simulink model "mod_torque_con_PID_Obs"  (R2023b)
settings: Solver=VariableStepAuto  StartTime=0.0  StopTime=20  MaxStep=1e-4  MinStep=1e-6  RelTol=1e-2
values from neighbouring files (symbols this model uses):
  alpha_Cu = 3.9e-3    (= 0.0039)    [analisis_estabilidad.m]    (also in parametros.m; parametros_sim.m)
  b_a = 0.0396    [parametros.m]
  b_eq = b_eq_max    (= 2.40277777778e-05)    [analisis_estabilidad.m]    (also in parametros.m = 2.19444444444e-05; parametros_sim.m = 2.19444444444e-05)
  b_m = 15.0e-6    (= 1.5e-05)    [analisis_estabilidad.m]    (also in parametros.m; parametros_sim.m)
  C_ts = 0.818    [analisis_estabilidad.m]    (also in parametros.m; parametros_sim.m)
  g = 9.80665    [analisis_estabilidad.m]    (also in parametros.m; parametros_sim.m)
  J_eq = J_eq_max    (= 4.58263888889e-05)    [analisis_estabilidad.m]    (also in parametros.m = 1.97847222222e-05; parametros_sim.m = 1.97847222222e-05)
  J_m = 14.0e-6    (= 1.4e-05)    [analisis_estabilidad.m]    (also in parametros.m; parametros_sim.m)
  k_l = (m*l_cm + m_l*l_l)*g    (= 2.4516625)    [analisis_estabilidad.m]    (also in parametros.m = 0.25; parametros_sim.m)
  K_sa = 31.656    [parametros.m]
  K_sia = 10129.78    [parametros.m]
  L_d = 6.6    [analisis_estabilidad.m]    (also in parametros.m = 0.0066; parametros_sim.m; polosyceros.m = L_d^3)
  L_ls = 0.8    [analisis_estabilidad.m]    (also in parametros.m = 0.0008; parametros_sim.m)
  L_q = 5.8    [analisis_estabilidad.m]    (also in parametros.m = 0.0058; parametros_sim.m; polosyceros.m = L_q^3)
  lambda_m = 0.016    [analisis_estabilidad.m]    (also in parametros.m; parametros_sim.m)
  P_p = 3    [analisis_estabilidad.m]    (also in parametros.m; parametros_sim.m)
  r = 120    [analisis_estabilidad.m]    (also in parametros.m; parametros_sim.m)
  R_s_ref = 1.02    [analisis_estabilidad.m]    (also in parametros.m; parametros_sim.m)
  R_ts_amb = 146.7    [analisis_estabilidad.m]    (also in parametros.m; parametros_sim.m)
  T_s_ref = 20    [analisis_estabilidad.m]    (also in parametros.m; parametros_sim.m)
undefined symbols (not defined in the file or in its folder): Ke_i, Ke_o2, Ke_omega, Ke_t2, Ke_theta, sat, tau, wn_mod, wnc, wnt, z
libraries: SignalEditorBlockLib x4
settings Model: Creator=AAgus  LastModifiedBy=Marti
settings SolverCC: MaxConsecutiveMinStep=100

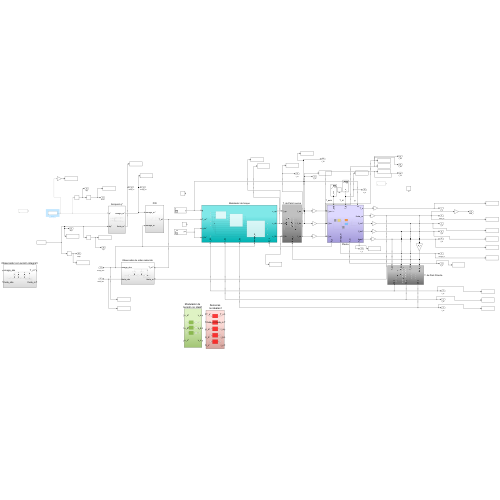
[thumbnail: Simulink's stored preview of the top-level diagram]
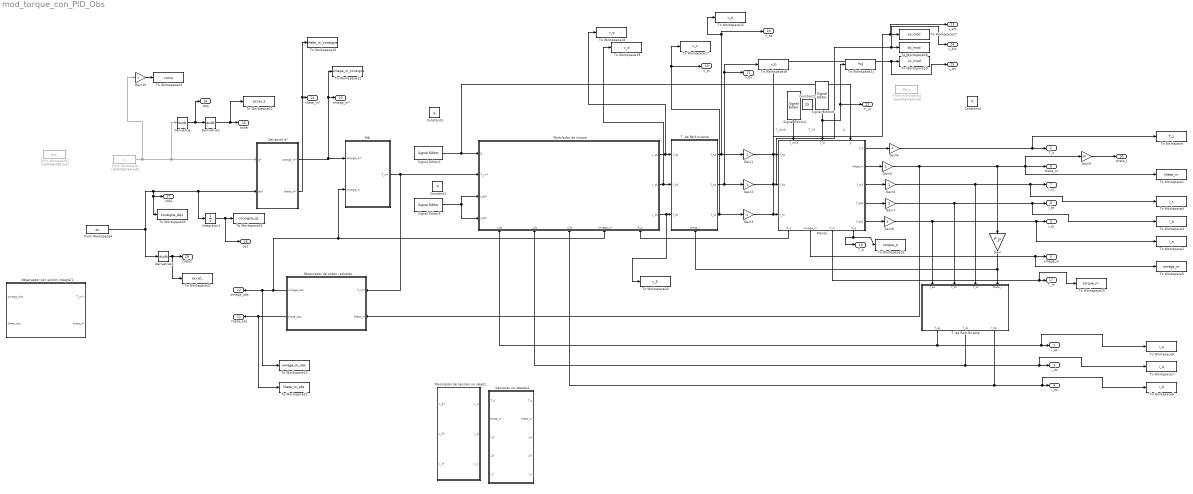
== system mod_torque_con_PID_Obs ==
  note: T_amb
  note: g
  note: T_ld
  Constant1 : Constant  Value=0
  Constant2 : Constant  Value=25
  Constant3 : Constant  Value=g
  Constant4 : Constant  Value=0
  Derivative : Derivative
  Derivative1 : Derivative
  Derivative3 : Derivative
  From Workspace : FromWorkspace  Commented=on  VariableName=u
  From Workspace1 : FromWorkspace  Commented=on  VariableName=duc
  From Workspace2 : FromWorkspace  Commented=on  VariableName=tld_c
  From Workspace4 : FromWorkspace  VariableName=du
  Gain : Gain  Gain=P_p
  Gain{1..8} (8 alike) : Gain
  Gain10 : Gain  Gain=r
  Gain9 : Gain  Gain=1/r
  Integrator1 : Integrator
  Modulador de tensión no ideal1 : Subsystem
  Modulador de torque : Subsystem
      settings: PortSchema="{\"entries\":[{\"content\":{\"sides\":[{\"content\":{\"connectorIds\":[\"In1\",\"In2\",\"In3\",\"In4\"]},\"type\":\"ConnectorPlacement.EquallySpacedRectSide\",\"uuid\":\"92ac8522-395f-4ce3-8f5e-792626a83240\"},{\"content\":{\"connectorIds\":[\"Out1\",\"Out2\",\"Out3\"],\"side\":\"RIGHT\"},\"type\":\"ConnectorPlacement.EquallySpacedRectSide\",\"uuid\":\"b1f2c717-a268-4393-91e6-df0d77a5b9df\"},{\"content\":{\"side\":\"TOP\"},\"type\":\"ConnectorPlacement.EquallySpacedRectSide\",\"uuid\":\"27380e77-d074-4889-aa22-28aab66abdda\"},{\"content\":{\"connectorIds\":[\"In5\",\"In6\",\"In7\",\"In8\",\"In9\"],\"side\":\"BOTTOM\"},\"type\":\"ConnectorPlacement.EquallySpacedRectSide\",\"uuid\":\"8a4427a4-2d74-404b-8b0d-69ab3b710b0e\"}]},\"type\":\"ConnectorPlacement.EquallySpacedConnector\",\"uuid\":\"19c0cced-0884-4633-8ad3-2d6d5d480879\"}],\"packageUris\":[\"http://schema.mathworks.com/mf0/Connector/R2020b\"],\"version\":\"1.0\"}"
  Observador con acción integral1 : Subsystem
      settings: PortSchema="{\"entries\":[{\"content\":{\"sides\":[{\"content\":{\"connectorIds\":[\"Out1\",\"Out2\"]},\"type\":\"ConnectorPlacement.EquallySpacedRectSide\",\"uuid\":\"7f1ab875-1cda-4cac-85ff-ce07181c17e4\"},{\"content\":{\"connectorIds\":[\"In1\",\"In2\"],\"side\":\"RIGHT\"},\"type\":\"ConnectorPlacement.EquallySpacedRectSide\",\"uuid\":\"6b91254d-cc96-42c9-a758-369a40099a6f\"},{\"content\":{\"side\":\"TOP\"},\"type\":\"ConnectorPlacement.EquallySpacedRectSide\",\"uuid\":\"4cd12954-6c23-434d-8bef-175e9edf0377\"}]},\"type\":\"ConnectorPlacement.EquallySpacedConnector\",\"uuid\":\"b17f3470-00fb-4a2f-9925-fdd3ec829801\"}],\"packageUris\":[\"http://schema.mathworks.com/mf0/Connector/R2020b\"],\"version\":\"1.0\"}"
  Observador de orden reducido : Subsystem
  PID : Subsystem
  Planta : Subsystem
      settings: PortSchema="{\"entries\":[{\"content\":{\"sides\":[{\"content\":{\"connectorIds\":[\"In1\",\"In2\",\"In3\"]},\"type\":\"ConnectorPlacement.EquallySpacedRectSide\",\"uuid\":\"9ff39df0-8326-46b1-b650-24ffd78ea64a\"},{\"content\":{\"connectorIds\":[\"Out1\",\"Out2\",\"Out3\",\"Out4\",\"Out5\"],\"side\":\"RIGHT\"},\"type\":\"ConnectorPlacement.EquallySpacedRectSide\",\"uuid\":\"3d3bc9f1-e392-438d-8ee1-0a3eb241c21d\"},{\"content\":{\"connectorIds\":[\"In4\",\"In5\",\"In6\"],\"side\":\"TOP\"},\"type\":\"ConnectorPlacement.EquallySpacedRectSide\",\"uuid\":\"c4910fb7-2fb9-4a3e-8c96-07515026454c\"},{\"content\":{\"connectorIds\":[\"Out6\",\"Out7\",\"Out8\",\"Out9\"],\"side\":\"BOTTOM\"},\"type\":\"ConnectorPlacement.EquallySpacedRectSide\",\"uuid\":\"63ebca1e-77c7-4a83-9d7f-f511e7e06496\"}]},\"type\":\"ConnectorPlacement.EquallySpacedConnector\",\"uuid\":\"6053906f-09a1-4145-a7f8-0fc1307cd3c1\"}],\"packageUris\":[\"http://schema.mathworks.com/mf0/Connector/R2020b\"],\"version\":\"1.0\"}"
  Sensores no ideales1 : Subsystem
  Set-point q* : Subsystem
  Signal Editor2 : SignalEditorBlockLib/Signal Editor  FileName=gravedad.mat  ActiveScenario=g  ActiveSignal=g  IsBus=off  OutputBusObjectStr=Bus: BusObject  SampleTime=0  Interpolate=off  ZeroCross=off  OutputAfterFinalValue=Setting to zero  Unit=inherit  PreserveSignalName=on  ApplySigPropsToAllScenarios=on  ApplySigPropsToAllSignals=off
  Signal Editor4 : SignalEditorBlockLib/Signal Editor  FileName=tamb.mat  ActiveScenario=T_amb  ActiveSignal=T_amb  IsBus=off  OutputBusObjectStr=Bus: BusObject  SampleTime=0  Interpolate=off  ZeroCross=off  OutputAfterFinalValue=Setting to zero  Unit=inherit  PreserveSignalName=on  ApplySigPropsToAllScenarios=on  ApplySigPropsToAllSignals=off
  Signal Editor5 : SignalEditorBlockLib/Signal Editor  FileName=corrientes_d0.mat  ActiveScenario=i_d0  ActiveSignal=i_d0  IsBus=off  OutputBusObjectStr=Bus: BusObject  SampleTime=0  Interpolate=off  ZeroCross=off  OutputAfterFinalValue=Setting to zero  Unit=inherit  PreserveSignalName=on  ApplySigPropsToAllScenarios=on  ApplySigPropsToAllSignals=off
  Signal Editor6 : SignalEditorBlockLib/Signal Editor  FileName=T_ld.mat  ActiveScenario=T_ld  ActiveSignal=T_ld  IsBus=off  OutputBusObjectStr=Bus: BusObject  SampleTime=0  Interpolate=off  ZeroCross=off  OutputAfterFinalValue=Setting to zero  Unit=inherit  PreserveSignalName=on  ApplySigPropsToAllScenarios=on  ApplySigPropsToAllSignals=off
  T. de Park Directa : Subsystem
  T. de Park Inversa : Subsystem
      settings: PortSchema="{\"entries\":[{\"content\":{\"sides\":[{\"content\":{\"connectorIds\":[\"In1\",\"In2\",\"In3\"]},\"type\":\"ConnectorPlacement.EquallySpacedRectSide\",\"uuid\":\"87a6b8c1-3fd8-4d15-81b7-6d19a59b6fe3\"},{\"content\":{\"connectorIds\":[\"Out1\",\"Out2\",\"Out3\"],\"side\":\"RIGHT\"},\"type\":\"ConnectorPlacement.EquallySpacedRectSide\",\"uuid\":\"ab7c1476-3519-4f3e-a604-adca334ac53f\"},{\"content\":{\"side\":\"TOP\"},\"type\":\"ConnectorPlacement.EquallySpacedRectSide\",\"uuid\":\"325a5f4a-a59c-4f4e-a8f9-a592ceecf271\"},{\"content\":{\"connectorIds\":[\"In4\"],\"side\":\"BOTTOM\"},\"type\":\"ConnectorPlacement.EquallySpacedRectSide\",\"uuid\":\"c8952c47-ee5f-4725-8e8a-36e5b1bf9c18\"}]},\"type\":\"ConnectorPlacement.EquallySpacedConnector\",\"uuid\":\"8a5a5c71-0ab4-4571-9e71-296ad9f443dc\"}],\"packageUris\":[\"http://schema.mathworks.com/mf0/Connector/R2020b\"],\"version\":\"1.0\"}"
  To Workspace : ToWorkspace  VariableName=T_s  SaveFormat=Timeseries  SampleTime=-1
  To Workspace1 : ToWorkspace  VariableName=theta_m  SaveFormat=Timeseries  SampleTime=-1
  To Workspace10 : ToWorkspace  VariableName=theta_m_consigna  SaveFormat=Timeseries  SampleTime=-1
  To Workspace11 : ToWorkspace  VariableName=omega_m_consigna  SaveFormat=Timeseries  SampleTime=-1
  To Workspace12 : ToWorkspace  VariableName=theta_m_obs  SaveFormat=Timeseries  SampleTime=-1
  To Workspace13 : ToWorkspace  VariableName=omega_m_obs  SaveFormat=Timeseries  SampleTime=-1
  To Workspace15 : ToWorkspace  VariableName=v_a  SaveFormat=Timeseries  SampleTime=-1
  To Workspace16 : ToWorkspace  VariableName=v_b  SaveFormat=Timeseries  SampleTime=-1
  To Workspace17 : ToWorkspace  VariableName=v_c  SaveFormat=Timeseries  SampleTime=-1
  To Workspace18 : ToWorkspace  VariableName=v_q  SaveFormat=Timeseries  SampleTime=-1
  To Workspace19 : ToWorkspace  VariableName=v_d  SaveFormat=Timeseries  SampleTime=-1
  To Workspace2 : ToWorkspace  VariableName=i_a  SaveFormat=Timeseries  SampleTime=-1
  To Workspace20 : ToWorkspace  VariableName=v_0  SaveFormat=Timeseries  SampleTime=-1
  To Workspace21 : ToWorkspace  VariableName=Tld  SaveFormat=Timeseries  SampleTime=-1
  To Workspace22 : ToWorkspace  VariableName=accel_1  SaveFormat=Timeseries  SampleTime=-1
  To Workspace24 : ToWorkspace  VariableName=comp  SaveFormat=Timeseries  SampleTime=-1
  To Workspace25 : ToWorkspace  VariableName=torque_m  SaveFormat=Timeseries  SampleTime=-1
  To Workspace26 : ToWorkspace  VariableName=torque_q  SaveFormat=Timeseries  SampleTime=-1
  To Workspace27 : ToWorkspace  VariableName=va_mod  SaveFormat=Timeseries  SampleTime=-1
  To Workspace28 : ToWorkspace  VariableName=vb_mod  SaveFormat=Timeseries  SampleTime=-1
  To Workspace29 : ToWorkspace  VariableName=vc_mod  SaveFormat=Timeseries  SampleTime=-1
  To Workspace3 : ToWorkspace  VariableName=i_b  SaveFormat=Timeseries  SampleTime=-1
  To Workspace30 : ToWorkspace  VariableName=consigna_dq1  SaveFormat=Timeseries  SampleTime=-1
  To Workspace31 : ToWorkspace  VariableName=accel_  SaveFormat=Timeseries  SampleTime=-1
  To Workspace32 : ToWorkspace  VariableName=consigna_q1  SaveFormat=Timeseries  SampleTime=-1
  To Workspace4 : ToWorkspace  VariableName=i_c  SaveFormat=Timeseries  SampleTime=-1
  To Workspace5 : ToWorkspace  VariableName=omega_m  SaveFormat=Timeseries  SampleTime=-1
  To Workspace6 : ToWorkspace  VariableName=i_0  SaveFormat=Timeseries  SampleTime=-1
  To Workspace7 : ToWorkspace  VariableName=i_d  SaveFormat=Timeseries  SampleTime=-1
  To Workspace8 : ToWorkspace  VariableName=i_q  SaveFormat=Timeseries  SampleTime=-1
  T_s : Outport
  i_qs : Outport  Port=2
  i_ds : Outport  Port=3
  i_0s : Outport  Port=4
  omega_m : Outport  Port=5
  theta_m : Outport  Port=6
  i_cs : Outport  Port=7
  i_bs : Outport  Port=8
  i_as : Outport  Port=9
  theta_l : Outport  Port=10
  theta_obs : Outport  Port=11
  omega_obs : Outport  Port=12
  omega_m* : Outport  Port=13
  theta_m* : Outport  Port=14
  accel : Outport  Port=15
  dqq : Outport  Port=16
  T_m : Outport  Port=17
  T_q : Outport  Port=18
  v_cs : Outport  Port=19
  v_as : Outport  Port=20
  v_bs : Outport  Port=21
  T_ld : Outport  Port=22
  v_am : Outport  Port=23
  v_bm : Outport  Port=24
  v_cm : Outport  Port=25
  cq1 : Outport  Port=26
  cdq1 : Outport  Port=27
  cddq1 : Outport  Port=28
  wires:
  Gain9/1 -> theta_l/1
  Gain7/1 -> To Workspace3/1, i_bs/1, T. de Park Directa/2(f_bs)
  Planta/2(theta_m) -> Gain5/1
  Signal Editor2/1 -> Modulador de torque/1(g), Planta/6(g)
  T. de Park Inversa/3(f_cs) -> Gain3/1, v_cs/1, To Workspace17/1
  Gain6/1 -> T. de Park Directa/3(f_cs), To Workspace4/1, i_cs/1
  Signal Editor4/1 -> Planta/4(T_amb)
  T. de Park Directa/2(f_ds) -> Modulador de torque/6(i_ds), To Workspace7/1, i_ds/1
  T. de Park Inversa/1(f_as) -> Gain1/1, v_as/1, To Workspace15/1
  Planta/4(f_bs1) -> Gain7/1
  T. de Park Directa/3(f_0s) -> To Workspace6/1, i_0s/1, Modulador de torque/7(i_0s)
  Planta/7(omega_m) -> To Workspace5/1, omega_m/1
  Gain4/1 -> To Workspace/1, T_s/1
  T. de Park Directa/1(f_qs) -> To Workspace8/1, i_qs/1, Modulador de torque/5(i_qs)
  T. de Park Inversa/2(f_bs) -> Gain2/1, To Workspace16/1, v_bs/1
  Gain5/1 -> Observador de orden reducido/2(theta_m), To Workspace1/1, Gain9/1, theta_m/1, Gain/1
  Planta/1(T_s) -> Gain4/1
  Gain8/1 -> To Workspace2/1, i_as/1, T. de Park Directa/1(f_as)
  Planta/3(f_cs1) -> Gain6/1
  Gain/1 -> T. de Park Directa/4(theta_r), T. de Park Inversa/4(theta_r)
  Planta/5(f_as1) -> Gain8/1
  Modulador de torque/1(v_qs) -> To Workspace18/1, T. de Park Inversa/1(f_qs)
  Modulador de torque/2(v_ds) -> To Workspace19/1, T. de Park Inversa/2(f_ds)
  Modulador de torque/3(v_0s) -> To Workspace20/1, T. de Park Inversa/3(f_0s)
  Planta/6(R_s) -> Modulador de torque/9(R_s)
  Signal Editor5/1 -> Modulador de torque/3(i_ds*), Modulador de torque/4(i_0s*)
  PID/1(T_m*) -> Observador de orden reducido/1(T_m'*), Modulador de torque/2(T_m'*)
  Set-point q*/1(omega_m*) -> omega_m*/1, To Workspace11/1, PID/1(omega_m*)
  Observador de orden reducido/2(theta_obs) -> To Workspace12/1, theta_obs/1
  Observador de orden reducido/1(omega_obs) -> PID/2(omega_m), Modulador de torque/8(omega_m), To Workspace13/1, omega_obs/1
  Set-point q*/2(theta_m*) -> To Workspace10/1, theta_m*/1
  From Workspace/1 -> Gain10/1, Derivative/1, Set-point q*/1(q*)
  Derivative/1 -> dqq/1, Derivative1/1
  Derivative1/1 -> To Workspace22/1, accel/1
  Gain10/1 -> To Workspace24/1
  Planta/8(T_m) -> To Workspace25/1, T_m/1
  Planta/9(T_q) -> T_q/1, To Workspace26/1
  Signal Editor6/1 -> To Workspace21/1, T_ld/1, Planta/5(T_ld)
  Gain1/1 -> v_am/1, To Workspace27/1, Planta/1(f_as)
  Gain2/1 -> v_bm/1, To Workspace28/1, Planta/2(f_bs)
  Gain3/1 -> v_cm/1, To Workspace29/1, Planta/3(f_cs)
  Derivative3/1 -> cddq1/1, To Workspace31/1
  Integrator1/1 -> To Workspace32/1, cq1/1
  From Workspace4/1 -> Derivative3/1, cdq1/1, To Workspace30/1, Set-point q*/2(dq*), Integrator1/1

== system mod_torque_con_PID_Obs/Modulador de tensión no ideal1 ==
  v_a* : Inport
  v_b* : Inport  Port=2
  v_c* : Inport  Port=3
  A : Subsystem
  B : Subsystem
  C : Subsystem
  Saturation3 : Saturate  UpperLimit=sat  LowerLimit=-sat
  Saturation4 : Saturate  UpperLimit=sat  LowerLimit=-sat
  Saturation5 : Saturate  UpperLimit=sat  LowerLimit=-sat
  v_a : Outport
  v_b : Outport  Port=2
  v_c : Outport  Port=3
  wires:
  Saturation5/1 -> v_c/1
  Saturation4/1 -> v_b/1
  Saturation3/1 -> v_a/1
  C/1(v_c) -> Saturation5/1
  B/1(v_b) -> Saturation4/1
  A/1(v_a) -> Saturation3/1
  v_b*/1 -> B/1(v_b*)
  v_a*/1 -> A/1(v_a*)
  v_c*/1 -> C/1(v_c*)

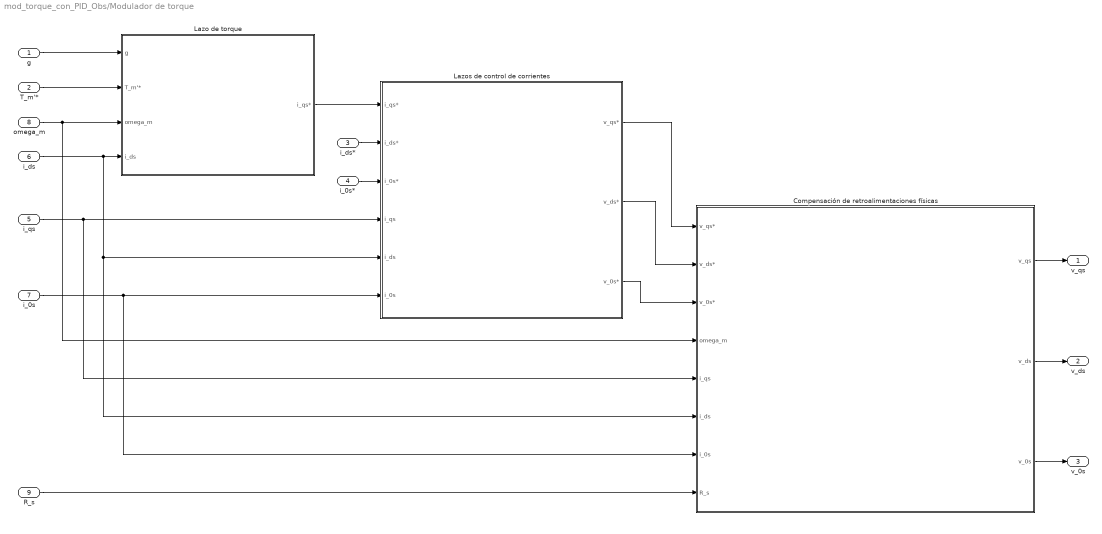
== system mod_torque_con_PID_Obs/Modulador de torque ==
  g : Inport
  T_m'* : Inport  Port=2
  i_ds* : Inport  Port=3
  i_0s* : Inport  Port=4
  i_qs : Inport  Port=5
  i_ds : Inport  Port=6
  i_0s : Inport  Port=7
  omega_m : Inport  Port=8
  R_s : Inport  Port=9
  Compensación de retroalimentaciones físicas : Subsystem
  Lazo de torque : Subsystem
  Lazos de control de corrientes : Subsystem
  v_qs : Outport
  v_ds : Outport  Port=2
  v_0s : Outport  Port=3
  wires:
  Lazos de control de corrientes/3(v_0s*) -> Compensación de retroalimentaciones físicas/3(v_0s*)
  i_ds*/1 -> Lazos de control de corrientes/2(i_ds*)
  T_m'*/1 -> Lazo de torque/2(T_m'*)
  Lazos de control de corrientes/1(v_qs*) -> Compensación de retroalimentaciones físicas/1(v_qs*)
  Lazos de control de corrientes/2(v_ds*) -> Compensación de retroalimentaciones físicas/2(v_ds*)
  omega_m/1 -> Lazo de torque/3(omega_m), Compensación de retroalimentaciones físicas/4(omega_m)
  Lazo de torque/1(i_qs*) -> Lazos de control de corrientes/1(i_qs*)
  g/1 -> Lazo de torque/1(g)
  Compensación de retroalimentaciones físicas/3(v_0s) -> v_0s/1
  i_ds/1 -> Compensación de retroalimentaciones físicas/6(i_ds), Lazos de control de corrientes/5(i_ds), Lazo de torque/4(i_ds)
  Compensación de retroalimentaciones físicas/1(v_qs) -> v_qs/1
  i_0s*/1 -> Lazos de control de corrientes/3(i_0s*)
  Compensación de retroalimentaciones físicas/2(v_ds) -> v_ds/1
  i_qs/1 -> Compensación de retroalimentaciones físicas/5(i_qs), Lazos de control de corrientes/4(i_qs)
  i_0s/1 -> Compensación de retroalimentaciones físicas/7(i_0s), Lazos de control de corrientes/6(i_0s)
  R_s/1 -> Compensación de retroalimentaciones físicas/8(R_s)

== system mod_torque_con_PID_Obs/Observador con acción integral1 ==
  note: e_theta
  T_m'* : Inport
  theta_m : Inport  Port=2
  Gain : Gain  Gain=1/J_eq
  Gain1 : Gain  Gain=Ke_o2
  Gain2 : Gain  Gain=Ke_i
  Gain3 : Gain  Gain=Ke_t2
  Integrator : Integrator
  Integrator1 : Integrator
  Integrator2 : Integrator
  Sum : Sum  Inputs=++|
  Sum1 : Sum  Inputs=++|
  Sum2 : Sum  Inputs=++|
  Sum3 : Sum  Inputs=+-
  omega_obs : Outport
  theta_obs : Outport  Port=2
  wires:
  Integrator/1 -> Sum2/2
  Sum/1 -> Sum1/2
  Gain1/1 -> Sum1/1
  Integrator2/1 -> Gain2/1
  Gain3/1 -> Sum2/1
  Sum2/1 -> Integrator1/1, omega_obs/1
  Integrator1/1 -> Sum3/2, theta_obs/1
  Gain2/1 -> Sum/1
  theta_m/1 -> Sum3/1
  T_m'*/1 -> Gain/1
  Gain/1 -> Sum/2
  Sum3/1 -> Gain3/1, Gain1/1, Integrator2/1
  Sum1/1 -> Integrator/1

== system mod_torque_con_PID_Obs/Observador de orden reducido ==
  note: e_theta
  T_m'* : Inport
  theta_m : Inport  Port=2
  Gain : Gain  Gain=1/J_eq
  Gain1 : Gain  Gain=Ke_omega
  Gain6 : Gain  Gain=Ke_theta
  Integrator : Integrator
  Integrator1 : Integrator
  Sum1 : Sum  Inputs=++|
  Sum3 : Sum  Inputs=++|
  Sum6 : Sum  Inputs=+-
  omega_obs : Outport
  theta_obs : Outport  Port=2
  wires:
  Gain/1 -> Sum1/2
  Sum1/1 -> Integrator/1
  Integrator1/1 -> theta_obs/1, Sum6/2
  theta_m/1 -> Sum6/1
  Gain6/1 -> Sum3/1
  Gain1/1 -> Sum1/1
  Sum6/1 -> Gain1/1, Gain6/1
  Sum3/1 -> omega_obs/1, Integrator1/1
  T_m'*/1 -> Gain/1
  Integrator/1 -> Sum3/2

== system mod_torque_con_PID_Obs/PID ==
  note: e_theta
  note: e_omega
  note: e_theta
  note: e_omega
  note: I
  note: P
  note: D
  omega_m* : Inport
  omega_m : Inport  Port=2
  Gain : Gain  Gain=K_sia
  Gain1 : Gain  Gain=K_sa
  Gain2 : Gain  Gain=b_a
  Integrator : Integrator
  Integrator1 : Integrator
  Sum : Sum  Inputs=|+-
  Sum1 : Sum  Inputs=+++
  T_m* : Outport
  wires:
  Gain2/1 -> Sum1/3
  Gain1/1 -> Sum1/2
  Integrator1/1 -> Gain1/1, Integrator/1
  Sum1/1 -> T_m*/1
  omega_m/1 -> Sum/2
  Gain/1 -> Sum1/1
  Integrator/1 -> Gain/1
  omega_m*/1 -> Sum/1
  Sum/1 -> Gain2/1, Integrator1/1

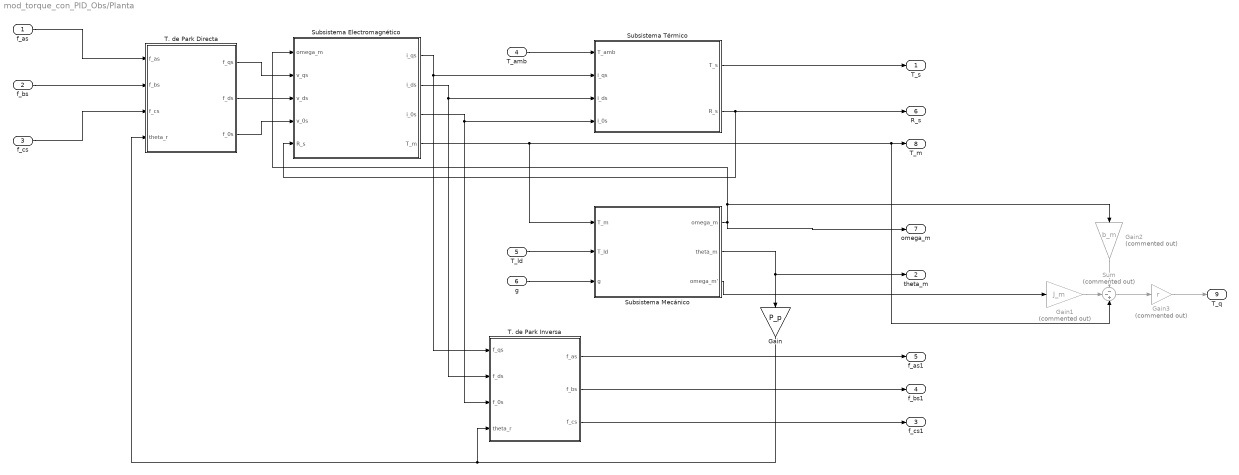
== system mod_torque_con_PID_Obs/Planta ==
  f_as : Inport
  f_bs : Inport  Port=2
  f_cs : Inport  Port=3
  T_amb : Inport  Port=4
  T_ld : Inport  Port=5
  g : Inport  Port=6
  Gain : Gain  Gain=P_p
  Gain1 : Gain  Commented=on  Gain=J_m
  Gain2 : Gain  Commented=on  Gain=b_m
  Gain3 : Gain  Commented=on  Gain=r
  Subsistema Electromagnético : Subsystem
  Subsistema Mecánico : Subsystem
  Subsistema Térmico : Subsystem
  Sum : Sum  Commented=on  Inputs=--+
  T. de Park Directa : Subsystem
  T. de Park Inversa : Subsystem
  T_s : Outport
  theta_m : Outport  Port=2
  f_cs1 : Outport  Port=3
  f_bs1 : Outport  Port=4
  f_as1 : Outport  Port=5
  R_s : Outport  Port=6
  omega_m : Outport  Port=7
  T_m : Outport  Port=8
  T_q : Outport  Port=9
  wires:
  f_as/1 -> T. de Park Directa/1(f_as)
  T. de Park Directa/1(f_qs) -> Subsistema Electromagnético/2(v_qs)
  T. de Park Directa/3(f_0s) -> Subsistema Electromagnético/4(v_0s)
  Subsistema Térmico/1(T_s) -> T_s/1
  T. de Park Inversa/1(f_as) -> f_as1/1
  T_amb/1 -> Subsistema Térmico/1(T_amb)
  Subsistema Electromagnético/3(i_0s) -> T. de Park Inversa/3(f_0s), Subsistema Térmico/4(i_0s)
  f_bs/1 -> T. de Park Directa/2(f_bs)
  T_ld/1 -> Subsistema Mecánico/2(T_ld)
  T. de Park Inversa/3(f_cs) -> f_cs1/1
  f_cs/1 -> T. de Park Directa/3(f_cs)
  T. de Park Inversa/2(f_bs) -> f_bs1/1
  Gain/1 -> T. de Park Directa/4(theta_r), T. de Park Inversa/4(theta_r)
  T. de Park Directa/2(f_ds) -> Subsistema Electromagnético/3(v_ds)
  Subsistema Térmico/2(R_s) -> Subsistema Electromagnético/5(R_s), R_s/1
  Subsistema Electromagnético/2(i_ds) -> T. de Park Inversa/2(f_ds), Subsistema Térmico/3(i_ds)
  Subsistema Electromagnético/1(i_qs) -> T. de Park Inversa/1(f_qs), Subsistema Térmico/2(i_qs)
  Subsistema Electromagnético/4(T_m) -> Sum/3, T_m/1, Subsistema Mecánico/1(T_m)
  Subsistema Mecánico/1(omega_m) -> omega_m/1, Gain2/1, Subsistema Electromagnético/1(omega_m)
  Subsistema Mecánico/2(theta_m) -> Gain/1, theta_m/1
  g/1 -> Subsistema Mecánico/3(g)
  Subsistema Mecánico/3(omega_m') -> Gain1/1
  Gain1/1 -> Sum/2
  Gain2/1 -> Sum/1
  Sum/1 -> Gain3/1
  Gain3/1 -> T_q/1

== system mod_torque_con_PID_Obs/Sensores no ideales1 ==
  T_s' : Inport
  theta_m' : Inport  Port=2
  i_a' : Inport  Port=3
  i_b' : Inport  Port=4
  i_c' : Inport  Port=5
  Sensor de Corriente A : Subsystem
  Sensor de Corriente B : Subsystem
  Sensor de Corriente C : Subsystem
  Sensor de Posición : Subsystem
  Sensor de Temperatura : Subsystem
  T_s : Outport
  theta_m : Outport  Port=2
  i_a : Outport  Port=3
  i_b : Outport  Port=4
  i_c : Outport  Port=5
  wires:
  i_c'/1 -> Sensor de Corriente C/1(i_c')
  i_b'/1 -> Sensor de Corriente B/1(i_b')
  Sensor de Corriente C/1(i_c) -> i_c/1
  Sensor de Temperatura/1(T_s) -> T_s/1
  theta_m'/1 -> Sensor de Posición/1(theta_m')
  i_a'/1 -> Sensor de Corriente A/1(i_a')
  Sensor de Corriente B/1(i_b) -> i_b/1
  Sensor de Posición/1(theta_m) -> theta_m/1
  T_s'/1 -> Sensor de Temperatura/1(T_s')
  Sensor de Corriente A/1(i_a) -> i_a/1

== system mod_torque_con_PID_Obs/Set-point q* ==
  q* : Inport
  dq* : Inport  Port=2
  Derivative : Derivative
  Gain1 : Gain  Gain=r
  Gain11 : Gain  Gain=r
  Integrator : Integrator
  Manual Switch : ManualSwitch  CurrentSetting=0
  Manual Switch1 : ManualSwitch  CurrentSetting=0
  omega_m* : Outport
  theta_m* : Outport  Port=2
  wires:
  q*/1 -> Gain11/1
  Gain11/1 -> Manual Switch/1, Derivative/1
  Manual Switch/1 -> theta_m*/1
  dq*/1 -> Gain1/1
  Manual Switch1/1 -> omega_m*/1
  Gain1/1 -> Manual Switch1/2, Integrator/1
  Derivative/1 -> Manual Switch1/1
  Integrator/1 -> Manual Switch/2

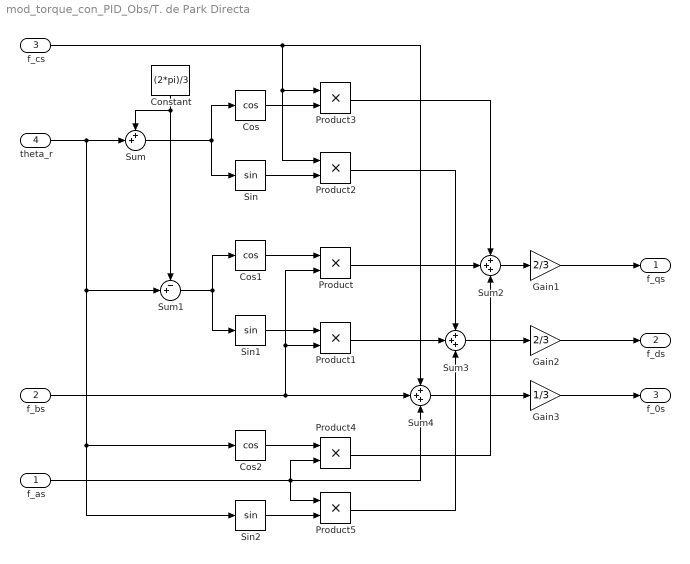
== system mod_torque_con_PID_Obs/T. de Park Directa ==
  f_as : Inport
  f_bs : Inport  Port=2
  f_cs : Inport  Port=3
  theta_r : Inport  Port=4
  Constant : Constant  Value=(2*pi)/3
  Cos : Trigonometry  Operator=cos
  Cos1 : Trigonometry  Operator=cos
  Cos2 : Trigonometry  Operator=cos
  Gain1 : Gain  Gain=2/3
  Gain2 : Gain  Gain=2/3
  Gain3 : Gain  Gain=1/3
  Product{,1..5} (6 alike) : Product
  Sin : Trigonometry
  Sin1 : Trigonometry
  Sin2 : Trigonometry
  Sum : Sum  Inputs=++|
  Sum1 : Sum  Inputs=-+|
  Sum2 : Sum  Inputs=+++
  Sum3 : Sum  Inputs=+++
  Sum4 : Sum  Inputs=+++
  f_qs : Outport
  f_ds : Outport  Port=2
  f_0s : Outport  Port=3
  wires:
  Product4/1 -> Sum2/3
  Cos1/1 -> Product/1
  theta_r/1 -> Sum/2, Sin2/1, Cos2/1, Sum1/2
  Sin1/1 -> Product1/1
  Sin2/1 -> Product5/2
  Product3/1 -> Sum2/1
  Cos2/1 -> Product4/1
  Product1/1 -> Sum3/2
  f_as/1 -> Sum4/3, Product4/2, Product5/1
  Sum2/1 -> Gain1/1
  Sum1/1 -> Sin1/1, Cos1/1
  f_bs/1 -> Sum4/2, Product/2, Product1/2
  Sum/1 -> Sin/1, Cos/1
  Product2/1 -> Sum3/1
  Sin/1 -> Product2/2
  Sum4/1 -> Gain3/1
  Gain1/1 -> f_qs/1
  f_cs/1 -> Sum4/1, Product2/1, Product3/1
  Gain2/1 -> f_ds/1
  Product/1 -> Sum2/2
  Sum3/1 -> Gain2/1
  Cos/1 -> Product3/2
  Constant/1 -> Sum1/1, Sum/1
  Gain3/1 -> f_0s/1
  Product5/1 -> Sum3/3

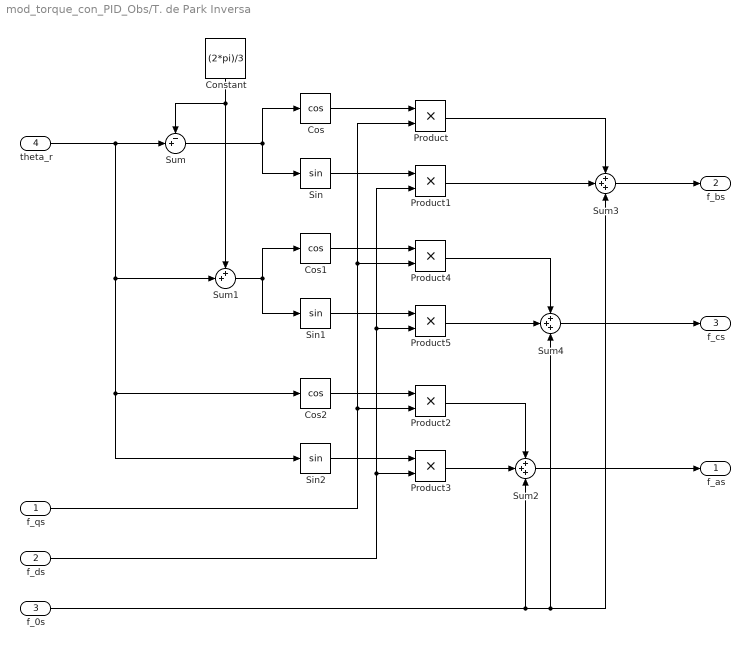
== system mod_torque_con_PID_Obs/T. de Park Inversa ==
  f_qs : Inport
  f_ds : Inport  Port=2
  f_0s : Inport  Port=3
  theta_r : Inport  Port=4
  Constant : Constant  Value=(2*pi)/3
  Cos : Trigonometry  Operator=cos
  Cos1 : Trigonometry  Operator=cos
  Cos2 : Trigonometry  Operator=cos
  Product{,1..5} (6 alike) : Product
  Sin : Trigonometry
  Sin1 : Trigonometry
  Sin2 : Trigonometry
  Sum : Sum  Inputs=-+|
  Sum1 : Sum  Inputs=++|
  Sum2 : Sum  Inputs=+++
  Sum3 : Sum  Inputs=+++
  Sum4 : Sum  Inputs=+++
  f_as : Outport
  f_bs : Outport  Port=2
  f_cs : Outport  Port=3
  wires:
  Product4/1 -> Sum4/1
  Sum2/1 -> f_as/1
  f_qs/1 -> Product4/2, Product/2, Product2/2
  Sum/1 -> Sin/1, Cos/1
  theta_r/1 -> Sum1/2, Cos2/1, Sin2/1, Sum/2
  Product1/1 -> Sum3/2
  Product3/1 -> Sum2/2
  Product5/1 -> Sum4/2
  Sin1/1 -> Product5/1
  Product/1 -> Sum3/1
  Cos/1 -> Product/1
  Sin2/1 -> Product3/1
  Cos1/1 -> Product4/1
  Sin/1 -> Product1/1
  f_0s/1 -> Sum3/3, Sum4/3, Sum2/3
  Sum3/1 -> f_bs/1
  Sum1/1 -> Sin1/1, Cos1/1
  Cos2/1 -> Product2/1
  Product2/1 -> Sum2/1
  Sum4/1 -> f_cs/1
  f_ds/1 -> Product3/2, Product5/2, Product1/2
  Constant/1 -> Sum/1, Sum1/1

== system mod_torque_con_PID_Obs/Modulador de tensión no ideal1/A ==
  note: y' = x2'
  note: x2 = x1'
  note: x1 = y
  v_a* : Inport
  Gain : Gain  Gain=wn_mod^2
  Gain1 : Gain  Gain=wn_mod
  Gain2 : Gain  Gain=z
  Gain3 : Gain  Gain=2
  Gain4 : Gain  Gain=wn_mod^2
  Integrator : Integrator
  Integrator1 : Integrator
  Sum : Sum  Inputs=+--
  v_a : Outport
  wires:
  Gain2/1 -> Gain3/1
  Gain1/1 -> Gain2/1
  v_a*/1 -> Gain/1
  Sum/1 -> Integrator/1
  Integrator1/1 -> v_a/1, Gain4/1
  Integrator/1 -> Gain1/1, Integrator1/1
  Gain/1 -> Sum/1
  Gain4/1 -> Sum/2
  Gain3/1 -> Sum/3

== system mod_torque_con_PID_Obs/Modulador de tensión no ideal1/B ==
  note: x1 = y
  note: x2 = x1'
  note: y' = x2'
  v_b* : Inport
  Gain : Gain  Gain=wn_mod^2
  Gain1 : Gain  Gain=wn_mod
  Gain2 : Gain  Gain=z
  Gain3 : Gain  Gain=2
  Gain4 : Gain  Gain=wn_mod^2
  Integrator : Integrator
  Integrator1 : Integrator
  Sum : Sum  Inputs=+--
  v_b : Outport
  wires:
  Gain3/1 -> Sum/3
  Gain4/1 -> Sum/2
  Gain/1 -> Sum/1
  Integrator/1 -> Integrator1/1, Gain1/1
  Integrator1/1 -> Gain4/1, v_b/1
  Sum/1 -> Integrator/1
  v_b*/1 -> Gain/1
  Gain1/1 -> Gain2/1
  Gain2/1 -> Gain3/1

== system mod_torque_con_PID_Obs/Modulador de tensión no ideal1/C ==
  note: y' = x2'
  note: x2 = x1'
  note: x1 = y
  v_c* : Inport
  Gain : Gain  Gain=wn_mod^2
  Gain1 : Gain  Gain=wn_mod
  Gain2 : Gain  Gain=z
  Gain3 : Gain  Gain=2
  Gain4 : Gain  Gain=wn_mod^2
  Integrator : Integrator
  Integrator1 : Integrator
  Sum : Sum  Inputs=+--
  v_c : Outport
  wires:
  Gain2/1 -> Gain3/1
  Gain1/1 -> Gain2/1
  v_c*/1 -> Gain/1
  Sum/1 -> Integrator/1
  Integrator1/1 -> v_c/1, Gain4/1
  Integrator/1 -> Gain1/1, Integrator1/1
  Gain/1 -> Sum/1
  Gain4/1 -> Sum/2
  Gain3/1 -> Sum/3

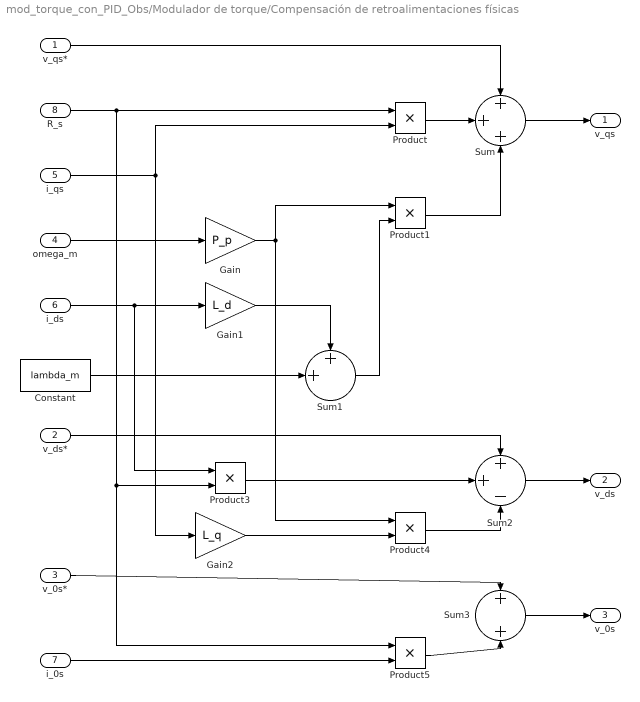
== system mod_torque_con_PID_Obs/Modulador de torque/Compensación de retroalimentaciones físicas ==
  v_qs* : Inport
  v_ds* : Inport  Port=2
  v_0s* : Inport  Port=3
  omega_m : Inport  Port=4
  i_qs : Inport  Port=5
  i_ds : Inport  Port=6
  i_0s : Inport  Port=7
  R_s : Inport  Port=8
  Constant : Constant  Value=lambda_m
  Gain : Gain  Gain=P_p
  Gain1 : Gain  Gain=L_d
  Gain2 : Gain  Gain=L_q
  Product{,1,3..5} (5 alike) : Product
  Sum : Sum  Inputs=+++
  Sum1 : Sum  Inputs=++|
  Sum2 : Sum  Inputs=++-
  Sum3 : Sum
  v_qs : Outport
  v_ds : Outport  Port=2
  v_0s : Outport  Port=3
  wires:
  v_qs*/1 -> Sum/1
  R_s/1 -> Product5/1, Product3/2, Product/1
  i_qs/1 -> Gain2/1, Product/2
  Product/1 -> Sum/2
  Product1/1 -> Sum/3
  omega_m/1 -> Gain/1
  Gain/1 -> Product4/1, Product1/1
  Sum1/1 -> Product1/2
  Gain1/1 -> Sum1/1
  i_ds/1 -> Product3/1, Gain1/1
  Constant/1 -> Sum1/2
  v_ds*/1 -> Sum2/1
  Product3/1 -> Sum2/2
  Gain2/1 -> Product4/2
  Product4/1 -> Sum2/3
  v_0s*/1 -> Sum3/1
  Product5/1 -> Sum3/2
  i_0s/1 -> Product5/2
  Sum/1 -> v_qs/1
  Sum2/1 -> v_ds/1
  Sum3/1 -> v_0s/1

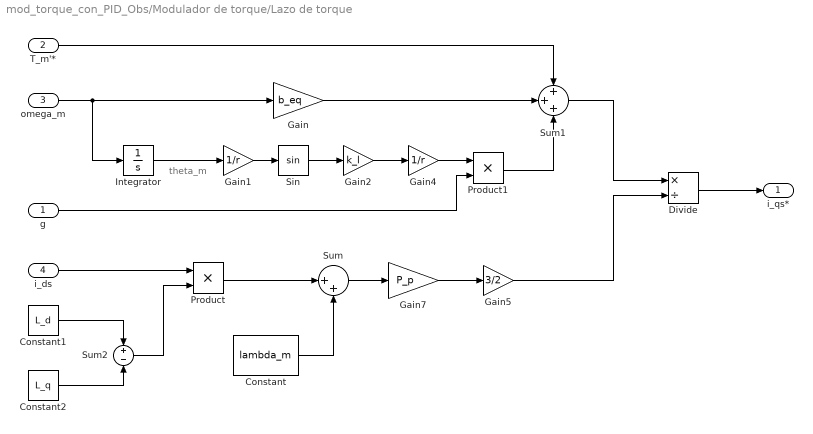
== system mod_torque_con_PID_Obs/Modulador de torque/Lazo de torque ==
  note: theta_m
  g : Inport
  T_m'* : Inport  Port=2
  omega_m : Inport  Port=3
  i_ds : Inport  Port=4
  Constant : Constant  Value=lambda_m
  Constant1 : Constant  Value=L_d
  Constant2 : Constant  Value=L_q
  Divide : Product  Inputs=*/
  Gain : Gain  Gain=b_eq
  Gain1 : Gain  Gain=1/r
  Gain2 : Gain  Gain=k_l
  Gain4 : Gain  Gain=1/r
  Gain5 : Gain  Gain=3/2
  Gain7 : Gain  Gain=P_p
  Integrator : Integrator
  Product : Product
  Product1 : Product
  Sin : Trigonometry
  Sum : Sum  Inputs=|++
  Sum1 : Sum  Inputs=+++
  Sum2 : Sum  Inputs=+-
  i_qs* : Outport
  wires:
  omega_m/1 -> Gain/1, Integrator/1
  Gain/1 -> Sum1/2
  Integrator/1 -> Gain1/1
  Gain1/1 -> Sin/1
  Product1/1 -> Sum1/3
  Sum1/1 -> Divide/1
  T_m'*/1 -> Sum1/1
  Divide/1 -> i_qs*/1
  Sin/1 -> Gain2/1
  Gain2/1 -> Gain4/1
  Gain7/1 -> Gain5/1
  Gain5/1 -> Divide/2
  Gain4/1 -> Product1/1
  g/1 -> Product1/2
  Sum/1 -> Gain7/1
  Constant/1 -> Sum/2
  Constant2/1 -> Sum2/2
  Constant1/1 -> Sum2/1
  Sum2/1 -> Product/2
  i_ds/1 -> Product/1
  Product/1 -> Sum/1

== system mod_torque_con_PID_Obs/Modulador de torque/Lazos de control de corrientes ==
  i_qs* : Inport
  i_ds* : Inport  Port=2
  i_0s* : Inport  Port=3
  i_qs : Inport  Port=4
  i_ds : Inport  Port=5
  i_0s : Inport  Port=6
  Gain : Gain  Gain=5000*L_q
  Gain1 : Gain  Gain=5000*L_d
  Gain2 : Gain  Gain=5000*L_ls
  Sum : Sum  Inputs=+-
  Sum1 : Sum  Inputs=+-
  Sum2 : Sum  Inputs=+-
  v_qs* : Outport
  v_ds* : Outport  Port=2
  v_0s* : Outport  Port=3
  wires:
  i_ds*/1 -> Sum1/1
  i_ds/1 -> Sum1/2
  i_qs/1 -> Sum/2
  Gain/1 -> v_qs*/1
  Sum2/1 -> Gain2/1
  i_0s/1 -> Sum2/2
  i_0s*/1 -> Sum2/1
  Sum/1 -> Gain/1
  Gain2/1 -> v_0s*/1
  i_qs*/1 -> Sum/1
  Sum1/1 -> Gain1/1
  Gain1/1 -> v_ds*/1

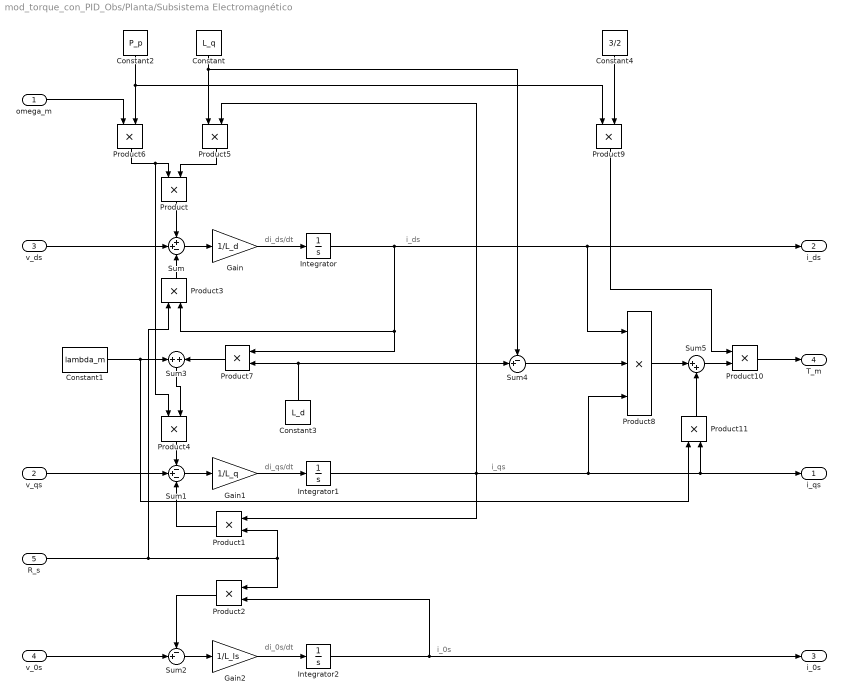
== system mod_torque_con_PID_Obs/Planta/Subsistema Electromagnético ==
  note: i_0s
  note: di_0s/dt
  note: i_qs
  note: i_ds
  note: di_ds/dt
  note: di_qs/dt
  omega_m : Inport
  v_qs : Inport  Port=2
  v_ds : Inport  Port=3
  v_0s : Inport  Port=4
  R_s : Inport  Port=5
  Constant : Constant  Value=L_q
  Constant1 : Constant  Value=lambda_m
  Constant2 : Constant  Value=P_p
  Constant3 : Constant  Value=L_d
  Constant4 : Constant  Value=3/2
  Gain : Gain  Gain=1/L_d
  Gain1 : Gain  Gain=1/L_q
  Gain2 : Gain  Gain=1/L_ls
  Integrator : Integrator
  Integrator1 : Integrator
  Integrator2 : Integrator
  Product{,1..7,9..11} (11 alike) : Product
  Product8 : Product  Inputs=3
  Sum : Sum  Inputs=++-
  Sum1 : Sum  Inputs=-+-
  Sum2 : Sum  Inputs=-+|
  Sum3 : Sum  Inputs=+|+
  Sum4 : Sum  Inputs=-+|
  Sum5 : Sum  Inputs=|++
  i_qs : Outport
  i_ds : Outport  Port=2
  i_0s : Outport  Port=3
  T_m : Outport  Port=4
  wires:
  Product4/1 -> Sum1/1
  Product1/1 -> Sum1/3
  Sum2/1 -> Gain2/1
  Product/1 -> Sum/1
  v_0s/1 -> Sum2/2
  v_qs/1 -> Sum1/2
  Gain2/1 -> Integrator2/1
  Product2/1 -> Sum2/1
  Integrator2/1 -> i_0s/1, Product2/2
  Integrator/1 -> Product8/1, i_ds/1, Product7/1, Product3/2
  Sum3/1 -> Product4/2
  Sum/1 -> Gain/1
  R_s/1 -> Product3/1, Product2/1, Product1/2
  Gain1/1 -> Integrator1/1
  Gain/1 -> Integrator/1
  Constant1/1 -> Product11/1, Sum3/1
  Product3/1 -> Sum/3
  Integrator1/1 -> Product8/3, Product11/2, i_qs/1, Product5/2, Product1/1
  Sum1/1 -> Gain1/1
  v_ds/1 -> Sum/2
  Constant/1 -> Sum4/1, Product5/1
  Product5/1 -> Product/2
  Constant2/1 -> Product9/1, Product6/2
  omega_m/1 -> Product6/1
  Product6/1 -> Product4/1, Product/1
  Product7/1 -> Sum3/2
  Constant3/1 -> Product7/2, Sum4/2
  Sum4/1 -> Product8/2
  Product8/1 -> Sum5/1
  Constant4/1 -> Product9/2
  Sum5/1 -> Product10/2
  Product9/1 -> Product10/1
  Product10/1 -> T_m/1
  Product11/1 -> Sum5/2

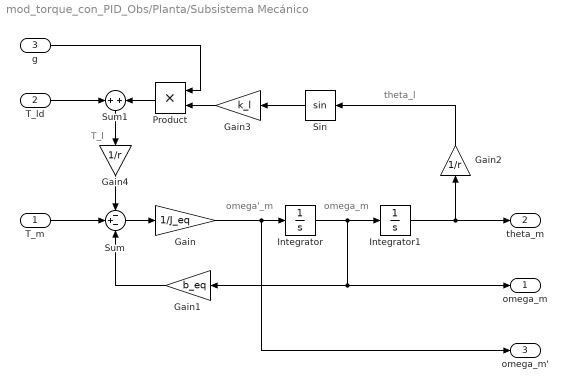
== system mod_torque_con_PID_Obs/Planta/Subsistema Mecánico ==
  note: theta_l
  note: omega'_m
  note: omega_m
  note: T_l
  T_m : Inport
  T_ld : Inport  Port=2
  g : Inport  Port=3
  Gain : Gain  Gain=1/J_eq
  Gain1 : Gain  Gain=b_eq
  Gain2 : Gain  Gain=1/r
  Gain3 : Gain  Gain=k_l
  Gain4 : Gain  Gain=1/r
  Integrator : Integrator
  Integrator1 : Integrator
  Product : Product
  Sin : Trigonometry
  Sum : Sum  Inputs=-+-
  Sum1 : Sum
  omega_m : Outport
  theta_m : Outport  Port=2
  omega_m' : Outport  Port=3
  wires:
  Gain3/1 -> Product/2
  Sin/1 -> Gain3/1
  Product/1 -> Sum1/2
  Integrator/1 -> Integrator1/1, Gain1/1, omega_m/1
  g/1 -> Product/1
  Integrator1/1 -> theta_m/1, Gain2/1
  T_ld/1 -> Sum1/1
  Gain/1 -> omega_m'/1, Integrator/1
  Sum1/1 -> Gain4/1
  Gain2/1 -> Sin/1
  Gain1/1 -> Sum/3
  T_m/1 -> Sum/2
  Sum/1 -> Gain/1
  Gain4/1 -> Sum/1

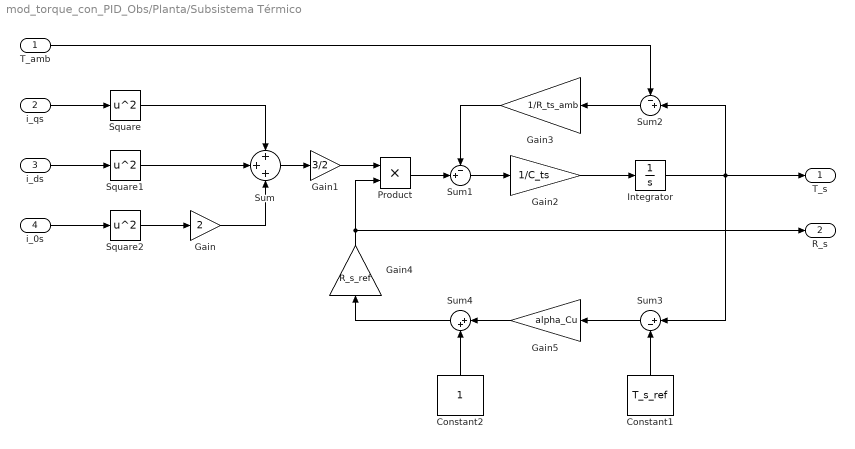
== system mod_torque_con_PID_Obs/Planta/Subsistema Térmico ==
  T_amb : Inport
  i_qs : Inport  Port=2
  i_ds : Inport  Port=3
  i_0s : Inport  Port=4
  Constant1 : Constant  Value=T_s_ref
  Constant2 : Constant
  Gain : Gain  Gain=2
  Gain1 : Gain  Gain=3/2
  Gain2 : Gain  Gain=1/C_ts
  Gain3 : Gain  Gain=1/R_ts_amb
  Gain4 : Gain  Gain=R_s_ref
  Gain5 : Gain  Gain=alpha_Cu
  Integrator : Integrator  InitialCondition=25
  Product : Product
  Square : Math  Operator=square
  Square1 : Math  Operator=square
  Square2 : Math  Operator=square
  Sum : Sum  Inputs=+++
  Sum1 : Sum  Inputs=-+|
  Sum2 : Sum  Inputs=-+|
  Sum3 : Sum  Inputs=|+-
  Sum4 : Sum  Inputs=|++
  T_s : Outport
  R_s : Outport  Port=2
  wires:
  Product/1 -> Sum1/2
  Gain1/1 -> Product/1
  Sum4/1 -> Gain4/1
  Sum3/1 -> Gain5/1
  Constant1/1 -> Sum3/2
  Sum2/1 -> Gain3/1
  Gain3/1 -> Sum1/1
  Sum1/1 -> Gain2/1
  i_ds/1 -> Square1/1
  Gain4/1 -> R_s/1, Product/2
  Gain2/1 -> Integrator/1
  Sum/1 -> Gain1/1
  Gain/1 -> Sum/3
  Square/1 -> Sum/1
  Square1/1 -> Sum/2
  Integrator/1 -> T_s/1, Sum2/2, Sum3/1
  Gain5/1 -> Sum4/1
  Square2/1 -> Gain/1
  i_0s/1 -> Square2/1
  Constant2/1 -> Sum4/2
  i_qs/1 -> Square/1
  T_amb/1 -> Sum2/1

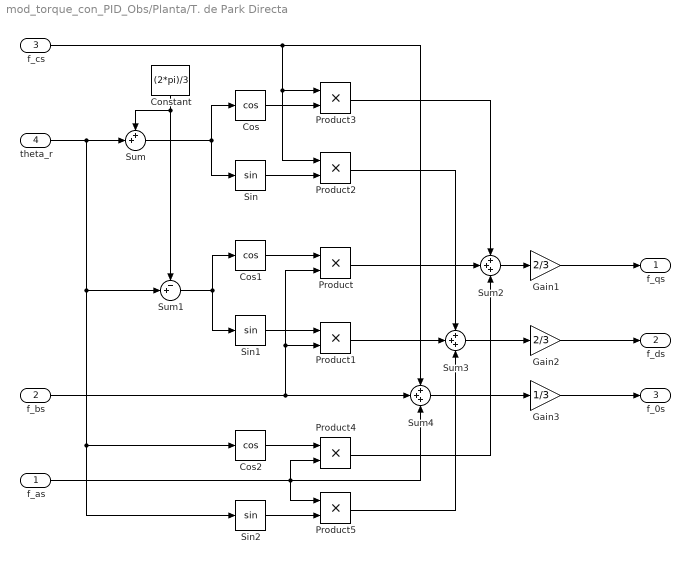
== system mod_torque_con_PID_Obs/Planta/T. de Park Directa ==
  f_as : Inport
  f_bs : Inport  Port=2
  f_cs : Inport  Port=3
  theta_r : Inport  Port=4
  Constant : Constant  Value=(2*pi)/3
  Cos : Trigonometry  Operator=cos
  Cos1 : Trigonometry  Operator=cos
  Cos2 : Trigonometry  Operator=cos
  Gain1 : Gain  Gain=2/3
  Gain2 : Gain  Gain=2/3
  Gain3 : Gain  Gain=1/3
  Product{,1..5} (6 alike) : Product
  Sin : Trigonometry
  Sin1 : Trigonometry
  Sin2 : Trigonometry
  Sum : Sum  Inputs=++|
  Sum1 : Sum  Inputs=-+|
  Sum2 : Sum  Inputs=+++
  Sum3 : Sum  Inputs=+++
  Sum4 : Sum  Inputs=+++
  f_qs : Outport
  f_ds : Outport  Port=2
  f_0s : Outport  Port=3
  wires:
  Product4/1 -> Sum2/3
  Cos1/1 -> Product/1
  theta_r/1 -> Sum/2, Sin2/1, Cos2/1, Sum1/2
  Sin1/1 -> Product1/1
  Sin2/1 -> Product5/2
  Product3/1 -> Sum2/1
  Cos2/1 -> Product4/1
  Product1/1 -> Sum3/2
  f_as/1 -> Sum4/3, Product4/2, Product5/1
  Sum2/1 -> Gain1/1
  Sum1/1 -> Sin1/1, Cos1/1
  f_bs/1 -> Sum4/2, Product/2, Product1/2
  Sum/1 -> Sin/1, Cos/1
  Product2/1 -> Sum3/1
  Sin/1 -> Product2/2
  Sum4/1 -> Gain3/1
  Gain1/1 -> f_qs/1
  f_cs/1 -> Sum4/1, Product2/1, Product3/1
  Gain2/1 -> f_ds/1
  Product/1 -> Sum2/2
  Sum3/1 -> Gain2/1
  Cos/1 -> Product3/2
  Constant/1 -> Sum1/1, Sum/1
  Gain3/1 -> f_0s/1
  Product5/1 -> Sum3/3

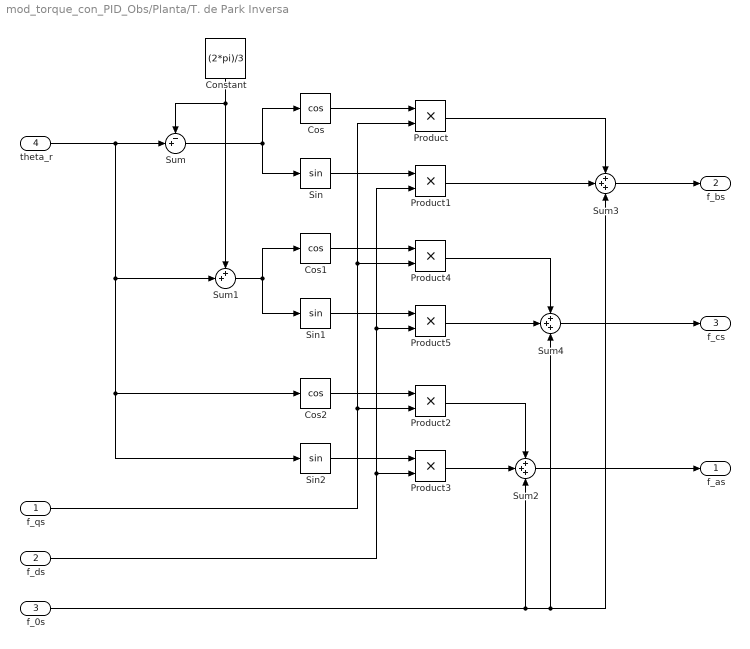
== system mod_torque_con_PID_Obs/Planta/T. de Park Inversa ==
  f_qs : Inport
  f_ds : Inport  Port=2
  f_0s : Inport  Port=3
  theta_r : Inport  Port=4
  Constant : Constant  Value=(2*pi)/3
  Cos : Trigonometry  Operator=cos
  Cos1 : Trigonometry  Operator=cos
  Cos2 : Trigonometry  Operator=cos
  Product{,1..5} (6 alike) : Product
  Sin : Trigonometry
  Sin1 : Trigonometry
  Sin2 : Trigonometry
  Sum : Sum  Inputs=-+|
  Sum1 : Sum  Inputs=++|
  Sum2 : Sum  Inputs=+++
  Sum3 : Sum  Inputs=+++
  Sum4 : Sum  Inputs=+++
  f_as : Outport
  f_bs : Outport  Port=2
  f_cs : Outport  Port=3
  wires:
  Product4/1 -> Sum4/1
  Sum2/1 -> f_as/1
  f_qs/1 -> Product4/2, Product/2, Product2/2
  Sum/1 -> Sin/1, Cos/1
  theta_r/1 -> Sum1/2, Cos2/1, Sin2/1, Sum/2
  Product1/1 -> Sum3/2
  Product3/1 -> Sum2/2
  Product5/1 -> Sum4/2
  Sin1/1 -> Product5/1
  Product/1 -> Sum3/1
  Cos/1 -> Product/1
  Sin2/1 -> Product3/1
  Cos1/1 -> Product4/1
  Sin/1 -> Product1/1
  f_0s/1 -> Sum3/3, Sum4/3, Sum2/3
  Sum3/1 -> f_bs/1
  Sum1/1 -> Sin1/1, Cos1/1
  Cos2/1 -> Product2/1
  Product2/1 -> Sum2/1
  Sum4/1 -> f_cs/1
  f_ds/1 -> Product3/2, Product5/2, Product1/2
  Constant/1 -> Sum/1, Sum1/1

== system mod_torque_con_PID_Obs/Sensores no ideales1/Sensor de Corriente A ==
  note: y' = x2'
  note: x2 = x1'
  note: x1 = y
  i_a' : Inport
  Gain : Gain  Gain=wnc^2
  Gain1 : Gain  Gain=wnc
  Gain2 : Gain  Gain=z
  Gain3 : Gain  Gain=2
  Gain4 : Gain  Gain=wnc^2
  Integrator : Integrator
  Integrator1 : Integrator
  Sum : Sum  Inputs=+--
  i_a : Outport
  wires:
  Gain2/1 -> Gain3/1
  Gain1/1 -> Gain2/1
  i_a'/1 -> Gain/1
  Sum/1 -> Integrator/1
  Integrator1/1 -> i_a/1, Gain4/1
  Integrator/1 -> Gain1/1, Integrator1/1
  Gain/1 -> Sum/1
  Gain4/1 -> Sum/2
  Gain3/1 -> Sum/3

== system mod_torque_con_PID_Obs/Sensores no ideales1/Sensor de Corriente B ==
  note: x1 = y
  note: x2 = x1'
  note: y' = x2'
  i_b' : Inport
  Gain : Gain  Gain=wnc^2
  Gain1 : Gain  Gain=wnc
  Gain2 : Gain  Gain=z
  Gain3 : Gain  Gain=2
  Gain4 : Gain  Gain=wnc^2
  Integrator : Integrator
  Integrator1 : Integrator
  Sum : Sum  Inputs=+--
  i_b : Outport
  wires:
  Gain3/1 -> Sum/3
  Gain4/1 -> Sum/2
  Gain/1 -> Sum/1
  Integrator/1 -> Integrator1/1, Gain1/1
  Integrator1/1 -> Gain4/1, i_b/1
  Sum/1 -> Integrator/1
  i_b'/1 -> Gain/1
  Gain1/1 -> Gain2/1
  Gain2/1 -> Gain3/1

== system mod_torque_con_PID_Obs/Sensores no ideales1/Sensor de Corriente C ==
  note: y' = x2'
  note: x2 = x1'
  note: x1 = y
  i_c' : Inport
  Gain : Gain  Gain=wnc^2
  Gain1 : Gain  Gain=wnc
  Gain2 : Gain  Gain=z
  Gain3 : Gain  Gain=2
  Gain4 : Gain  Gain=wnc^2
  Integrator : Integrator
  Integrator1 : Integrator
  Sum : Sum  Inputs=+--
  i_c : Outport
  wires:
  Gain2/1 -> Gain3/1
  Gain1/1 -> Gain2/1
  i_c'/1 -> Gain/1
  Sum/1 -> Integrator/1
  Integrator1/1 -> i_c/1, Gain4/1
  Integrator/1 -> Gain1/1, Integrator1/1
  Gain/1 -> Sum/1
  Gain4/1 -> Sum/2
  Gain3/1 -> Sum/3

== system mod_torque_con_PID_Obs/Sensores no ideales1/Sensor de Posición ==
  note: x1 = y
  note: x2 = x1'
  note: y' = x2'
  theta_m' : Inport
  Gain : Gain  Gain=wnt^2
  Gain1 : Gain  Gain=wnt
  Gain2 : Gain  Gain=z
  Gain3 : Gain  Gain=2
  Gain4 : Gain  Gain=wnt^2
  Integrator : Integrator
  Integrator1 : Integrator
  Sum : Sum  Inputs=+--
  theta_m : Outport
  wires:
  Gain3/1 -> Sum/3
  Gain4/1 -> Sum/2
  Gain/1 -> Sum/1
  Integrator/1 -> Integrator1/1, Gain1/1
  Integrator1/1 -> Gain4/1, theta_m/1
  Sum/1 -> Integrator/1
  theta_m'/1 -> Gain/1
  Gain1/1 -> Gain2/1
  Gain2/1 -> Gain3/1

== system mod_torque_con_PID_Obs/Sensores no ideales1/Sensor de Temperatura ==
  T_s' : Inport
  Gain : Gain  Gain=1/tau
  Integrator : Integrator  InitialCondition=25
  Sum : Sum  Inputs=|+-
  T_s : Outport
  wires:
  T_s'/1 -> Sum/1
  Gain/1 -> Integrator/1
  Sum/1 -> Gain/1
  Integrator/1 -> Sum/2, T_s/1
